simulink model "CONTROLLED_6_pulse_rectifier"  (R2013a)
settings: Solver=ode45  StartTime=0.0  StopTime=0.06  RelTol=1e-3
libraries: powerlib x16, powerlib_meascontrol x1, dspstat3 x1
settings Model: Creator=hp  LastModifiedBy=hp

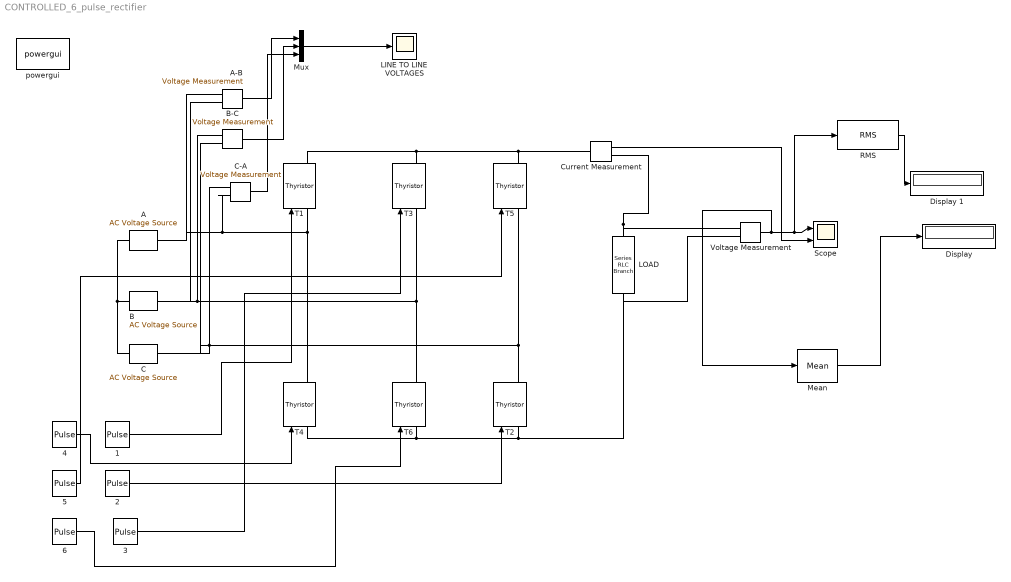
== system CONTROLLED_6_pulse_rectifier ==
  " LOAD" : powerlib/Elements/Series RLC Branch  LConnTagsString=__new0  RConnTagsString=__new0  BranchType=R  Resistance=10  Inductance=50e-2  SetiL0=off  InitialCurrent=0  Capacitance=1e-6  Setx0=off  InitialVoltage=0  Measurements=None
  1 : DiscretePulseGenerator  PulseType=Time based  Amplitude=5  Period=0.02  PulseWidth=5  PhaseDelay=(0.02/360)*30
  2 : DiscretePulseGenerator  PulseType=Time based  Amplitude=5  Period=0.02  PulseWidth=5  PhaseDelay=(0.02/360)*90
  3 : DiscretePulseGenerator  PulseType=Time based  Amplitude=5  Period=0.02  PulseWidth=5  PhaseDelay=(0.02/360)*150
  4 : DiscretePulseGenerator  PulseType=Time based  Amplitude=5  Period=0.02  PulseWidth=5  PhaseDelay=(0.02/360)*210
  5 : DiscretePulseGenerator  PulseType=Time based  Amplitude=5  Period=0.02  PulseWidth=5  PhaseDelay=(0.02/360)*270
  6 : DiscretePulseGenerator  PulseType=Time based  Amplitude=5  Period=0.02  PulseWidth=5  PhaseDelay=(0.02/360)*330
  A : powerlib/Electrical Sources/AC Voltage Source  Amplitude=312  Phase=0  Frequency=50  SampleTime=0  Measurements=None
  A-B : powerlib/Measurements/Voltage Measurement  PhasorSimulation=off  OutputType=Complex  PSBequivalent=0
  B : powerlib/Electrical Sources/AC Voltage Source  Amplitude=312  Phase=-120  Frequency=50  SampleTime=0  Measurements=None
  B-C : powerlib/Measurements/Voltage Measurement  PhasorSimulation=off  OutputType=Complex  PSBequivalent=0
  C : powerlib/Electrical Sources/AC Voltage Source  Amplitude=312  Phase=120  Frequency=50  SampleTime=0  Measurements=None
  C-A : powerlib/Measurements/Voltage Measurement  PhasorSimulation=off  OutputType=Complex  PSBequivalent=0
  Current Measurement : powerlib/Measurements/Current Measurement  PhasorSimulation=off  OutputType=Complex  PSBequivalent=0
  Display : Display
  Display 1 : Display
  LINE TO LINE VOLTAGES : Scope
      settings: TimeRange=0.1  YMin=-600  YMax=600  SaveName=line_voltage1
  Mean : powerlib_meascontrol/Measurements/Mean  Freq=60  Vinit=0  Ts=0
  Mux : Mux  Inputs=3
  RMS : dspstat3/RMS  run=off  reset_popup=None  InputProcessing=Columns as channels (frame based)  directionMode=Each column  dimension=1  treatSBRowAsCol=on
  Scope : Scope  NumInputPorts=2
      settings: TimeRange=0.1  YMin=-5~-5  YMax=5~5
  T{1..6} (6 alike) : powerlib/Power Electronics/Thyristor  Ron=0.001  Lon=0  Vf=0.8  IC=0  Rs=500  Cs=250e-9  Measurements=on
  Voltage Measurement : powerlib/Measurements/Voltage Measurement  PhasorSimulation=off  OutputType=Complex  PSBequivalent=0
  powergui : powerlib/powergui  Priority=1  SimulationMode=Continuous  SolverType=Tustin  SampleTime=50e-6  frequency=60  SPID=off  DisableSnubberDevices=off  DisableRonSwitches=off  DisableVfSwitches=off  SwTol=0  Interpol=off  DisplayEquations=off  frequencyindice=50  Pbase=100e6  ErrMax=1e-4  Iterations=50  UnitsV=kV  UnitsW=MW  FunctionMessages=off  echomessages=off  HookPort=off  EnableUseOfTLC=off  x0status=blocks  RestoreLinks=warning  ResistiveCurrentMeasurement=off  Frange=[0:2:500]  Ylog=off  Xlog=on  ShowGrid=off  save=off  variable=ZData  ZoomFFT=off  StartTime=0.0  cycles=1  DisplayStyle=1  fundamental=60  FreqAxis=off  MaxFrequency=1000  frequencyindicesteady=1  RmsSteady=1  display=off  Ts=0  methode=off
  wires:
  A-B/1 -> Mux/1
  B-C/1 -> Mux/2
  C-A/1 -> Mux/3
  1/1 -> T1/1
  2/1 -> T2/1
  3/1 -> T3/1
  4/1 -> T4/1
  5/1 -> T5/1
  6/1 -> T6/1
  Voltage Measurement/1 -> Mean/1, RMS/1, Scope/1
  Current Measurement/1 -> Scope/2
  Mux/1 -> LINE TO LINE VOLTAGES/1
  Mean/1 -> Display/1
  RMS/1 -> Display 1/1
  connections:
  A/LConn1 -- C/LConn1 -- B/LConn1
  T5/LConn1 -- C/RConn1 -- B-C/LConn2 -- C-A/LConn1 -- T2/RConn1
  T3/LConn1 -- B-C/LConn1 -- A-B/LConn2 -- B/RConn1 -- T6/RConn1
  T1/LConn1 -- C-A/LConn2 -- A/RConn1 -- A-B/LConn1 -- T4/RConn1
  T1/RConn1 -- T3/RConn1 -- Current Measurement/LConn1 -- T5/RConn1
  T4/LConn1 -- T6/LConn1 -- Voltage Measurement/LConn2 -- " LOAD"/LConn1 -- T2/LConn1
  Current Measurement/RConn1 -- Voltage Measurement/LConn1 -- " LOAD"/RConn1
